simulink model "nonlinearCarModel"  (R2017a)
settings: Solver=ode45  StartTime=0.0  StopTime=simulation_time  MaxStep=0.1  RelTol=1e-3
values from neighbouring files (symbols this model uses):
  B_c = 1/car_tire_rad    (= 3.59712230216)    [initialization.m]
  C_c = aero_c    (= 0.07455105)    [initialization.m]
  car_tire_rad = 0.556/2    (= 0.278)    [initialization.m]
  D_c = car_mass*gravity    (= 1569.6)    [initialization.m]
  drivetrain_loss = 0.95    [initialization.m]
  Gr_1 = 15    [initialization.m]
  Gr_2 = 15    [initialization.m]
  Ki_m1 = 100*Motor1.resistance    [initialization.m]
  Ki_m2 = 100*Motor2.resistance    [initialization.m]
  Ki_vel = 0.00015    [initialization.m]
  Kp_m1 = 100*Motor1.inductance    [initialization.m]
  Kp_m2 = 100*Motor2.inductance    [initialization.m]
  Kp_vel = 1700    [initialization.m]
  m1_volt_limit = 48    [initialization.m]
  m2_volt_limit = 48    [initialization.m]
  M_c = car_mass + car_tire_inertia    (= 170.558459707)    [initialization.m]
  Motor1 = Re50    [initialization.m]
  Motor2 = Re50    [initialization.m]
  N_c = car_roll_friction    (= 2.04048)    [initialization.m]
  smooth_angle_track = [0 1 2 3 4 5 6 7 8 9 10 11 ... (3320 elements, 1660x2)]    [track_angles.mat]
libraries: fuzblock x3, simulink x3
settings Model: Creator=jorgejac  LastModifiedBy=FF

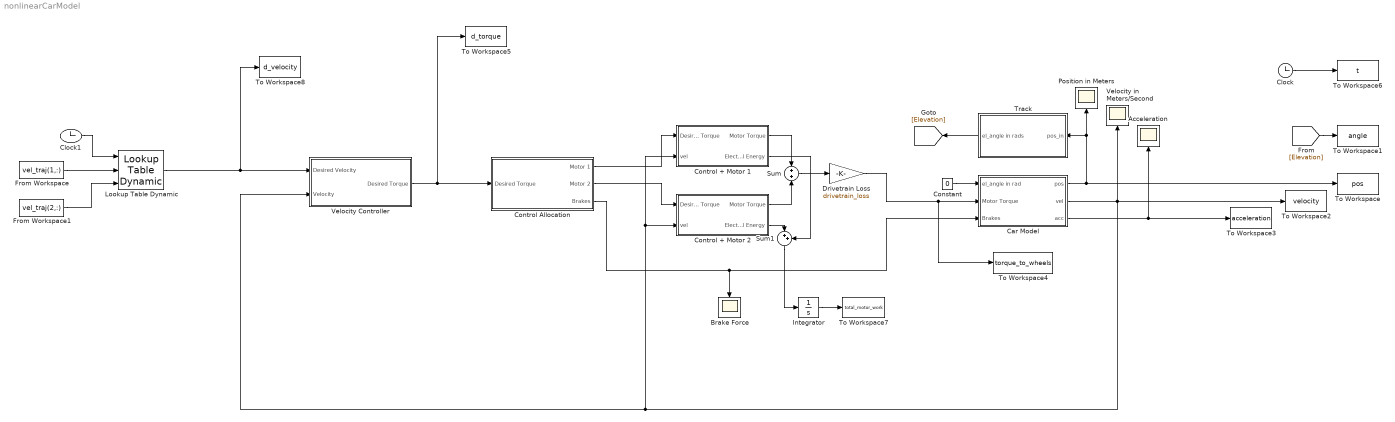
== system nonlinearCarModel ==
  Acceleration : Scope
  Brake Force : Scope
  Car Model : Subsystem
  Clock : Clock
  Clock1 : Clock
  Constant : Constant  Value=0
  Control + Motor 1 : Subsystem
  Control + Motor 2 : Subsystem
  Control Allocation : Subsystem
  Drivetrain Loss : Gain  Gain=drivetrain_loss
  From Workspace : FromWorkspace  VariableName=vel_traj(1,:)  SampleTime=0  Interpolate=off  OutputAfterFinalValue=Holding final value
  From Workspace1 : FromWorkspace  VariableName=vel_traj(2,:)  SampleTime=0  Interpolate=off  OutputAfterFinalValue=Holding final value
  Integrator : Integrator
  Lookup Table Dynamic : simulink/Lookup Tables/Lookup Table Dynamic  LookUpMeth=Interpolation-Use End Values  OutDataType=fixdt('double')  OutScaling=[]  OutputDataTypeScalingMode=Specify via dialog  OutDataTypeStr=double  DoSatur=off
      settings: SourceProductName=Simulink
  Position in Meters : Scope
  Sum : Sum  Inputs=+|+
  Sum1 : Sum  Inputs=|++
  To Workspace : ToWorkspace  VariableName=pos  SampleTime=-1
  To Workspace1 : ToWorkspace  VariableName=angle  SampleTime=-1
  To Workspace2 : ToWorkspace  VariableName=velocity  SampleTime=-1
  To Workspace3 : ToWorkspace  VariableName=acceleration  SampleTime=-1
  To Workspace4 : ToWorkspace  VariableName=torque_to_wheels  SampleTime=-1
  To Workspace5 : ToWorkspace  VariableName=d_torque  SampleTime=-1
  To Workspace6 : ToWorkspace  VariableName=t  SampleTime=-1
  To Workspace7 : ToWorkspace  VariableName=total_motor_work  SampleTime=-1
  To Workspace8 : ToWorkspace  VariableName=d_velocity  SampleTime=-1
  Track : Subsystem
  Velocity Controller : Subsystem
  Velocity in Meters/Second : Scope
  wires:
  Car Model/1(pos) -> To Workspace/1, Position in Meters/1, Track/1(pos_in)
  [Elevation] -> To Workspace1/1
  Clock/1 -> To Workspace6/1
  Car Model/3(acc) -> Acceleration/1, To Workspace3/1
  Car Model/2(vel) -> Control + Motor 1/2(vel), Control + Motor 2/2(vel), Velocity Controller/2(Velocity), To Workspace2/1, Velocity in Meters/Second/1
  Track/1("el_angle in rads ") -> [Elevation]
  Velocity Controller/1(Desired Torque) -> To Workspace5/1, Control Allocation/1("Desired Torque ")
  Constant/1 -> Car Model/1(el_angle in rad)
  Control Allocation/2("Motor 2 ") -> Control + Motor 2/1(Desired Torque)
  Control + Motor 1/1(Motor Torque) -> Sum/1
  Control + Motor 2/1(Motor Torque) -> Sum/2
  Integrator/1 -> To Workspace7/1
  Control + Motor 2/2(Electrical Energy) -> Sum1/1
  Control + Motor 1/2(Electrical Energy) -> Sum1/2
  Sum1/1 -> Integrator/1
  Control Allocation/1("Motor 1 ") -> Control + Motor 1/1(Desired Torque)
  Sum/1 -> Drivetrain Loss/1
  Drivetrain Loss/1 -> To Workspace4/1, Car Model/2(Motor Torque)
  Lookup Table Dynamic/1 -> To Workspace8/1, Velocity Controller/1(Desired Velocity)
  From Workspace/1 -> Lookup Table Dynamic/2
  From Workspace1/1 -> Lookup Table Dynamic/3
  Clock1/1 -> Lookup Table Dynamic/1
  Control Allocation/3(Brakes) -> Brake Force/1, Car Model/3(Brakes)

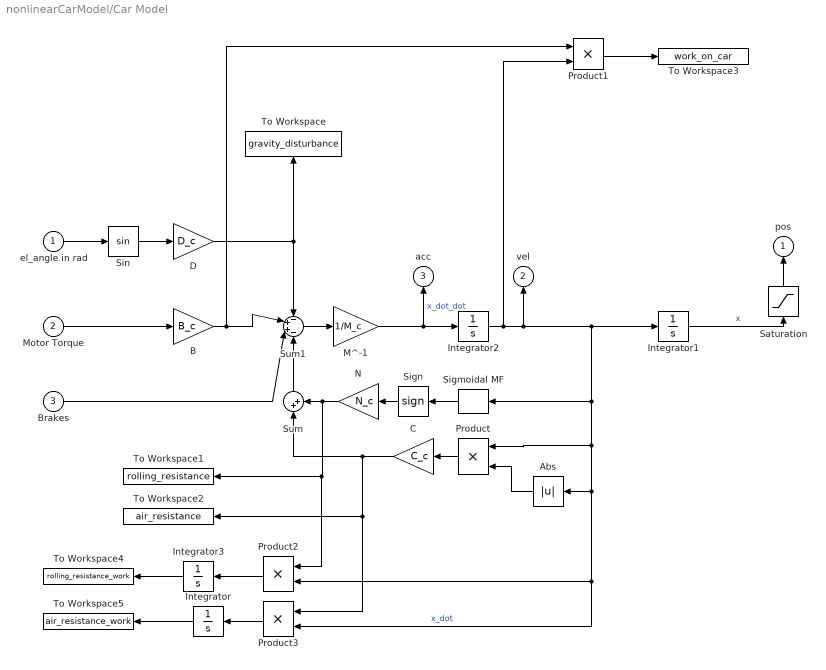
== system nonlinearCarModel/Car Model ==
  el_angle in rad : Inport
  Motor Torque : Inport  Port=2
  Brakes : Inport  Port=3
  Abs : Abs
  B : Gain  Gain=B_c
  C : Gain  Gain=C_c
  D : Gain  Gain=D_c
  Integrator{,1..3} (4 alike) : Integrator
  M^-1 : Gain  Gain=1/M_c
  N : Gain  Gain=N_c
  Product{,1..3} (4 alike) : Product
  Saturation : Saturate  UpperLimit=inf  LowerLimit=0
  Sigmoidal MF : fuzblock/Membership  Functions/Sigmoidal MF  a=0.001  c=0
      settings: SourceProductName=Fuzzy Logic Toolbox  SourceProductBaseCode=FL
  Sign : Signum
  Sin : Trigonometry
  Sum : Sum  Inputs=|++
  Sum1 : Sum  Inputs=-++-
  To Workspace : ToWorkspace  VariableName=gravity_disturbance  SampleTime=-1
  To Workspace1 : ToWorkspace  VariableName=rolling_resistance  SampleTime=-1
  To Workspace2 : ToWorkspace  VariableName=air_resistance  SampleTime=-1
  To Workspace3 : ToWorkspace  VariableName=work_on_car  SampleTime=-1
  To Workspace4 : ToWorkspace  VariableName=rolling_resistance_work  SampleTime=-1
  To Workspace5 : ToWorkspace  VariableName=air_resistance_work  SampleTime=-1
  pos : Outport
  vel : Outport  Port=2
  acc : Outport  Port=3
  wires:
  M^-1/1 -> Integrator2/1, acc/1  "x_dot_dot"
  Integrator1/1 -> Saturation/1  "x"
  Integrator2/1 -> Product1/2, Integrator1/1, Sigmoidal MF/1, Product/1, Product3/2, Product2/2, Abs/1, vel/1  "x_dot"
  Product/1 -> C/1
  N/1 -> Product2/1, To Workspace1/1, Sum/2
  C/1 -> Product3/1, To Workspace2/1, Sum/1
  Sum/1 -> Sum1/4
  Sum1/1 -> M^-1/1
  B/1 -> Sum1/2, Product1/1
  Motor Torque/1 -> B/1
  Sin/1 -> D/1
  el_angle in rad/1 -> Sin/1
  D/1 -> To Workspace/1, Sum1/1
  Sign/1 -> N/1
  Sigmoidal MF/1 -> Sign/1
  Product1/1 -> To Workspace3/1
  Saturation/1 -> pos/1
  Abs/1 -> Product/2
  Product2/1 -> Integrator3/1
  Product3/1 -> Integrator/1
  Brakes/1 -> Sum1/3
  Integrator/1 -> To Workspace5/1
  Integrator3/1 -> To Workspace4/1

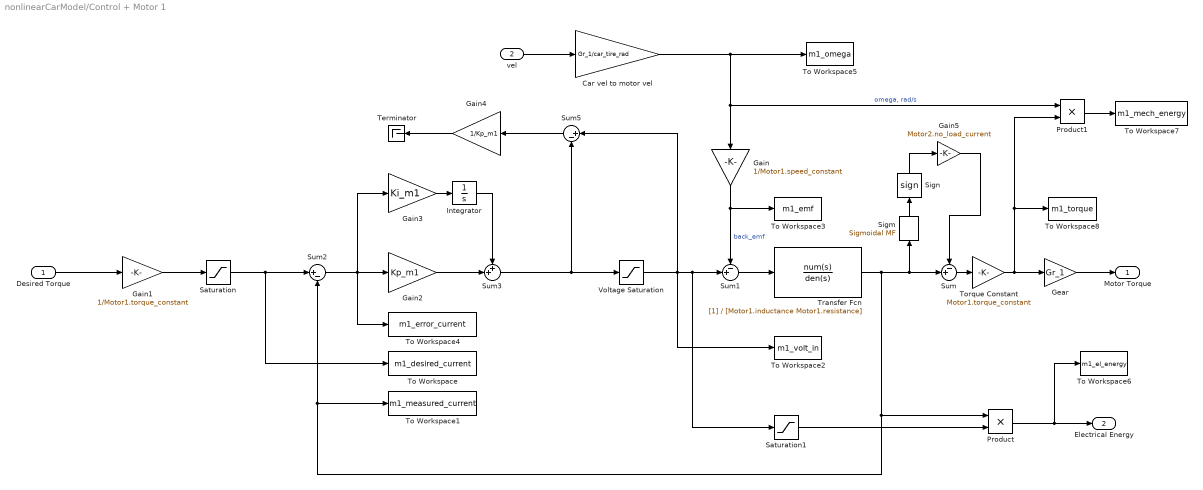
== system nonlinearCarModel/Control + Motor 1 ==
  Desired Torque : Inport
  vel : Inport  Port=2
  Car vel to motor vel : Gain  Gain=Gr_1/car_tire_rad
  Gain : Gain  Gain=1/Motor1.speed_constant
  Gain1 : Gain  Gain=1/Motor1.torque_constant
  Gain2 : Gain  Gain=Kp_m1
  Gain3 : Gain  Gain=Ki_m1
  Gain4 : Gain  Gain=1/Kp_m1
  Gain5 : Gain  Gain=Motor2.no_load_current
  Gear : Gain  Gain=Gr_1
  Integrator : Integrator
  Product : Product
  Product1 : Product
  Saturation : Saturate  UpperLimit=Motor1.max_current  LowerLimit=-Motor2.max_current
  Saturation1 : Saturate  UpperLimit=m1_volt_limit  LowerLimit=0
  Sigm : fuzblock/Membership  Functions/Sigmoidal MF  a=0.001  c=0
      settings: SourceProductName=Fuzzy Logic Toolbox  SourceProductBaseCode=FL
  Sign : Signum
  Sum : Sum  Inputs=-+|
  Sum1 : Sum  Inputs=-+|
  Sum2 : Sum  Inputs=|+-
  Sum3 : Sum  Inputs=++|
  Sum5 : Sum  Inputs=|+-
  Terminator : Terminator
  To Workspace : ToWorkspace  VariableName=m1_desired_current  SampleTime=-1
  To Workspace1 : ToWorkspace  VariableName=m1_measured_current  SampleTime=-1
  To Workspace2 : ToWorkspace  VariableName=m1_volt_in  SampleTime=-1
  To Workspace3 : ToWorkspace  VariableName=m1_emf  SampleTime=-1
  To Workspace4 : ToWorkspace  VariableName=m1_error_current  SampleTime=-1
  To Workspace5 : ToWorkspace  VariableName=m1_omega  SampleTime=-1
  To Workspace6 : ToWorkspace  VariableName=m1_el_energy  SampleTime=-1
  To Workspace7 : ToWorkspace  VariableName=m1_mech_energy  SampleTime=-1
  To Workspace8 : ToWorkspace  VariableName=m1_torque  SampleTime=-1
  Torque Constant : Gain  Gain=Motor1.torque_constant
  Transfer Fcn : TransferFcn  Denominator=[Motor1.inductance Motor1.resistance]
  Voltage Saturation : Saturate  UpperLimit=m1_volt_limit  LowerLimit=0
  Motor Torque : Outport
  Electrical Energy : Outport  Port=2
  wires:
  Sum1/1 -> Transfer Fcn/1
  vel/1 -> Car vel to motor vel/1
  Car vel to motor vel/1 -> Gain/1, Product1/1, To Workspace5/1  "omega, rad/s"
  Gain/1 -> Sum1/1, To Workspace3/1  "back_emf"
  Desired Torque/1 -> Gain1/1
  Gain1/1 -> Saturation/1
  Sum/1 -> Torque Constant/1
  Gain2/1 -> Sum3/2
  Sum3/1 -> Voltage Saturation/1, Sum5/2
  Integrator/1 -> Sum3/1
  Sum5/1 -> Gain4/1
  Gear/1 -> Motor Torque/1
  Gain3/1 -> Integrator/1
  Sum2/1 -> Gain3/1, To Workspace4/1, Gain2/1
  Saturation/1 -> Sum2/1, To Workspace/1
  Product/1 -> To Workspace6/1, Electrical Energy/1
  Voltage Saturation/1 -> To Workspace2/1, Sum5/1, Saturation1/1, Sum1/2
  Product1/1 -> To Workspace7/1
  Torque Constant/1 -> Gear/1, To Workspace8/1, Product1/2
  Gain4/1 -> Terminator/1
  Transfer Fcn/1 -> Product/1, To Workspace1/1, Sum2/2, Sigm/1, Sum/2
  Sigm/1 -> Sign/1
  Sign/1 -> Gain5/1
  Gain5/1 -> Sum/1
  Saturation1/1 -> Product/2

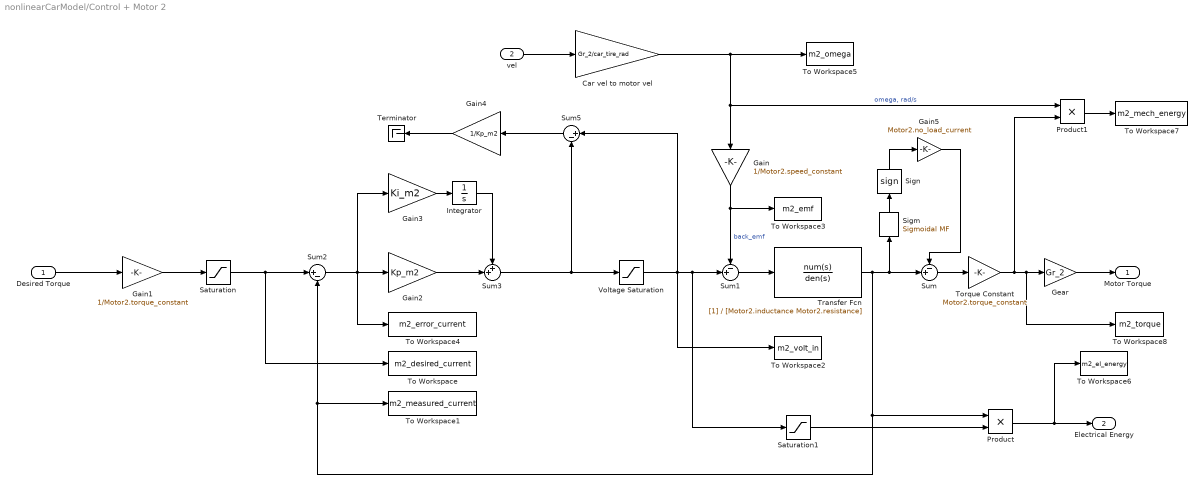
== system nonlinearCarModel/Control + Motor 2 ==
  Desired Torque : Inport
  vel : Inport  Port=2
  Car vel to motor vel : Gain  Gain=Gr_2/car_tire_rad
  Gain : Gain  Gain=1/Motor2.speed_constant
  Gain1 : Gain  Gain=1/Motor2.torque_constant
  Gain2 : Gain  Gain=Kp_m2
  Gain3 : Gain  Gain=Ki_m2
  Gain4 : Gain  Gain=1/Kp_m2
  Gain5 : Gain  Gain=Motor2.no_load_current
  Gear : Gain  Gain=Gr_2
  Integrator : Integrator
  Product : Product
  Product1 : Product
  Saturation : Saturate  UpperLimit=Motor2.max_current  LowerLimit=-Motor2.max_current
  Saturation1 : Saturate  UpperLimit=m2_volt_limit  LowerLimit=0
  Sigm : fuzblock/Membership  Functions/Sigmoidal MF  a=0.001  c=0
      settings: SourceProductName=Fuzzy Logic Toolbox  SourceProductBaseCode=FL
  Sign : Signum
  Sum : Sum  Inputs=-+|
  Sum1 : Sum  Inputs=-+|
  Sum2 : Sum  Inputs=|+-
  Sum3 : Sum  Inputs=++|
  Sum5 : Sum  Inputs=|+-
  Terminator : Terminator
  To Workspace : ToWorkspace  VariableName=m2_desired_current  SampleTime=-1
  To Workspace1 : ToWorkspace  VariableName=m2_measured_current  SampleTime=-1
  To Workspace2 : ToWorkspace  VariableName=m2_volt_in  SampleTime=-1
  To Workspace3 : ToWorkspace  VariableName=m2_emf  SampleTime=-1
  To Workspace4 : ToWorkspace  VariableName=m2_error_current  SampleTime=-1
  To Workspace5 : ToWorkspace  VariableName=m2_omega  SampleTime=-1
  To Workspace6 : ToWorkspace  VariableName=m2_el_energy  SampleTime=-1
  To Workspace7 : ToWorkspace  VariableName=m2_mech_energy  SampleTime=-1
  To Workspace8 : ToWorkspace  VariableName=m2_torque  SampleTime=-1
  Torque Constant : Gain  Gain=Motor2.torque_constant
  Transfer Fcn : TransferFcn  Denominator=[Motor2.inductance Motor2.resistance]
  Voltage Saturation : Saturate  UpperLimit=m2_volt_limit  LowerLimit=0
  Motor Torque : Outport
  Electrical Energy : Outport  Port=2
  wires:
  Gain5/1 -> Sum/1
  Sum1/1 -> Transfer Fcn/1
  vel/1 -> Car vel to motor vel/1
  Car vel to motor vel/1 -> Gain/1, Product1/1, To Workspace5/1  "omega, rad/s"
  Gain/1 -> Sum1/1, To Workspace3/1  "back_emf"
  Desired Torque/1 -> Gain1/1
  Gain1/1 -> Saturation/1
  Sum/1 -> Torque Constant/1
  Gain2/1 -> Sum3/2
  Sum3/1 -> Voltage Saturation/1, Sum5/2
  Integrator/1 -> Sum3/1
  Sum5/1 -> Gain4/1
  Gear/1 -> Motor Torque/1
  Gain3/1 -> Integrator/1
  Sum2/1 -> Gain3/1, To Workspace4/1, Gain2/1
  Saturation/1 -> Sum2/1, To Workspace/1
  Product/1 -> To Workspace6/1, Electrical Energy/1
  Voltage Saturation/1 -> To Workspace2/1, Sum5/1, Saturation1/1, Sum1/2
  Product1/1 -> To Workspace7/1
  Torque Constant/1 -> To Workspace8/1, Gear/1, Product1/2
  Gain4/1 -> Terminator/1
  Transfer Fcn/1 -> Sigm/1, Sum/2, Product/1, To Workspace1/1, Sum2/2
  Sigm/1 -> Sign/1
  Sign/1 -> Gain5/1
  Saturation1/1 -> Product/2

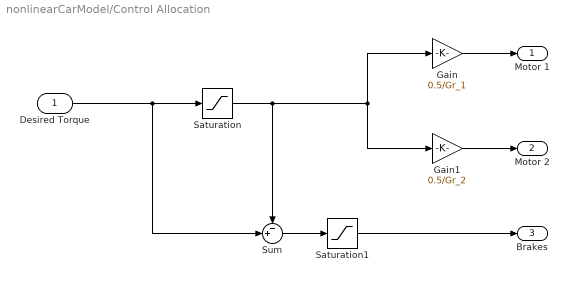
== system nonlinearCarModel/Control Allocation ==
  "Desired Torque " : Inport
  Gain : Gain  Gain=0.5/Gr_1
  Gain1 : Gain  Gain=0.5/Gr_2
  Saturation : Saturate  UpperLimit=Motor1.max_current*Gr_1*Motor1.torque_constant*2  LowerLimit=-Motor1.max_current*Gr_1*Motor1.torque_constant*2
  Saturation1 : Saturate  UpperLimit=0  LowerLimit=-1700
  Sum : Sum  Inputs=-+|
  "Motor 1 " : Outport
  "Motor 2 " : Outport  Port=2
  Brakes : Outport  Port=3
  wires:
  Gain/1 -> "Motor 1 "/1
  Gain1/1 -> "Motor 2 "/1
  "Desired Torque "/1 -> Sum/2, Saturation/1
  Saturation/1 -> Gain/1, Gain1/1, Sum/1
  Sum/1 -> Saturation1/1
  Saturation1/1 -> Brakes/1

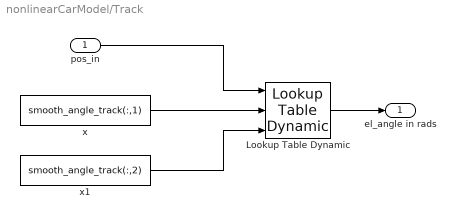
== system nonlinearCarModel/Track ==
  pos_in : Inport
  Lookup Table Dynamic : simulink/Lookup Tables/Lookup Table Dynamic  LookUpMeth=Interpolation-Use End Values  OutDataType=fixdt('double')  OutScaling=[]  OutputDataTypeScalingMode=Specify via dialog  OutDataTypeStr=double  DoSatur=off
      settings: SourceProductName=Simulink
  x : Constant  Value=smooth_angle_track(:,1)
  x1 : Constant  Value=smooth_angle_track(:,2)  VectorParams1D=off
  "el_angle in rads " : Outport
  wires:
  pos_in/1 -> Lookup Table Dynamic/1
  Lookup Table Dynamic/1 -> "el_angle in rads "/1
  x1/1 -> Lookup Table Dynamic/3
  x/1 -> Lookup Table Dynamic/2

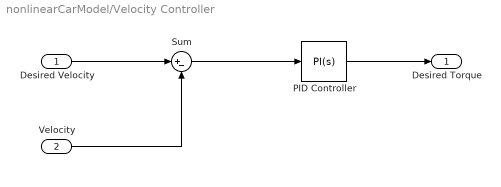
== system nonlinearCarModel/Velocity Controller ==
  Desired Velocity : Inport
  Velocity : Inport  Port=2
  PID Controller : simulink/Continuous/PID Controller  Controller=PI  TimeDomain=Continuous-time  SampleTime=-1  IntegratorMethod=Forward Euler  FilterMethod=Forward Euler  Form=Parallel  UseFilter=on  ControllerParametersSource=internal  P=Kp_vel  I=Ki_vel  D=83  N=2081  InitialConditionSource=internal  InitialConditionForIntegrator=0  InitialConditionForFilter=0  ExternalReset=none  LimitOutput=off  UpperSaturationLimit=45  LowerSaturationLimit=-inf  LinearizeAsGain=on  AntiWindupMode=none  Kb=1  TrackingMode=off  Kt=1  PParamMin=[]  PParamMax=[]  IParamMin=[]  IParamMax=[]  DParamMin=[]  DParamMax=[]  NParamMin=[]  NParamMax=[]  KbParamMin=[]  KbParamMax=[]  KtParamMin=[]  KtParamMax=[]  POutMin=[]  POutMax=[]  IOutMin=[]  IOutMax=[]  DOutMin=[]  DOutMax=[]  NOutMin=[]  NOutMax=[]  KbOutMin=[]  KbOutMax=[]  KtOutMin=[]  KtOutMax=[]  IntegratorOutMin=[]  IntegratorOutMax=[]  FilterOutMin=[]  FilterOutMax=[]  SumOutMin=[]  SumOutMax=[]  SumI1OutMin=[]  SumI1OutMax=[]  SumI2OutMin=[]  SumI2OutMax=[]  SumI3OutMin=[]  SumI3OutMax=[]  SumDOutMin=[]  SumDOutMax=[]  SaturationOutMin=[]  SaturationOutMax=[]  IntegratorContinuousStateAttributes=''  IntegratorStateMustResolveToSignalObject=off  IntegratorRTWStateStorageClass=Auto  FilterContinuousStateAttributes=''  FilterStateMustResolveToSignalObject=off  FilterRTWStateStorageClass=Auto  DifferentiatorICPrevScaledInput=0  DifferentiatorOutMin=[]  DifferentiatorOutMax=[]  InitialConditionSetting=State (most efficient)
  Sum : Sum  Inputs=|+-
  Desired Torque : Outport
  wires:
  PID Controller/1 -> Desired Torque/1
  Desired Velocity/1 -> Sum/1
  Sum/1 -> PID Controller/1
  Velocity/1 -> Sum/2
